simulink library "simplex_lib"  (R2020b)
settings: Solver=VariableStepAuto  StartTime=0.0  StopTime=10.0  RelTol=1e-3
values from neighbouring files (symbols this model uses):
  Ts = 1/Fs    [MainSimulink.m]
undefined symbols (not defined in the file or in its folder): ang_r, DiscIntNeverNeededParam, P_dc, Sbase, Tm_pu, Vbase, w0, Wbase, wbase
libraries: powerlib x62, $bdroot x14
settings Model: Creator=admin_user  LastModifiedBy=admin_user
settings DataIOCC: ReturnWorkspaceOutputs=off
settings DebuggingCC: ArithmeticOperatorsInVariantConditions=warning
settings SFSimCC: SimUseLocalCustomCode=off  CustomCodeUndefinedFunction=UseInterfaceOnly
settings RTWCC: RTWUseLocalCustomCode=off

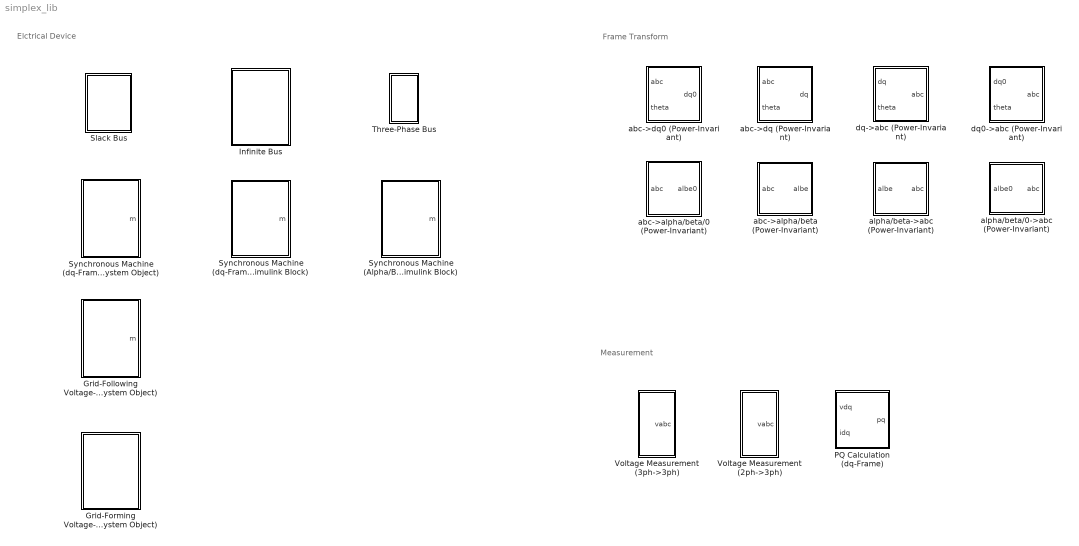
== system simplex_lib ==
  note: Elctrical Device
  note: Measurement
  note: Frame Transform
  Grid-Following Voltage-Source Inverter (dq-Frame System Object) : Subsystem  mask{Sbase=Sbase, Vbase=Vbase, Wbase=Wbase, Ts=Ts, DeviceType=10, DevicePara=[], PowerFlow=[], x0=[0; 0; 0; 0; 2.5*Vbase; 0; 0; Wbase; 0], OtherInputs=[ang_r; P_dc]}
      mask prompts: Ts "Ts (s)"
  Grid-Forming Voltage-Source Inverter (dq-Frame System Object) : Subsystem  mask{DeviceType=10, DevicePara=[], PowerFlow=[], theta0=0, ang_r=0, P_dc=0, Ts=Ts, x0=[0;0;0;0;1;0;0;0;0;0;w0;1]}
      mask prompts: Ts "Ts (s)"
  Infinite Bus : Subsystem  mask{Sbase=1, Vbase=1, Wbase=Wbase, Vdq0=[1,0,0], w=1, theta0=0}
      mask prompts: Sbase "Sbase (VA)"; Vbase "Vbase (V)"; Wbase "Wbase (rad/s)"; Vdq0 "Vdq0 (pu)"; w "w (pu)"; theta0 "theta0 (rad)"
  PQ Calculation (dq-Frame) : Subsystem  mask{wfil=wbase/10, Ts=Ts}
      mask prompts: wfil "Filter Bandwidth (rad/s)"; Ts "Sampling Time"
  Slack Bus : Subsystem  mask{vd=1, vq=0, v0=0, w=1, theta0=0, Vbase=Vbase, Wbase=Wbase}
      mask prompts: vd "vd (pu)"; vq "vq (pu)"; v0 "v0 (pu)"; w "w (pu)"; theta0 "theta0 (rad)"; Vbase "Vbase (V)"; Wbase "Wbase (rad/s)"
  Synchronous Machine (Alpha/Beta-Frame Simulink Block) : Subsystem  mask{Ts=Ts, Sbase=Sbase, Vbase=Vbase, Wbase=Wbase, R=0.01, L=0.3, J=2*3.5, D=10, psi_f=1.1229, Tm=-10.890, w0=1, theta0=0}
      mask prompts: Ts "Sampling Time, Ts (s)"; Sbase "Base Power, Sbase (VA)"; Vbase "Base Voltage, Vbase (V)"; Wbase "Base Angular Frequency, Wbase (rad/s)"; R "Stator Resistance, R (pu)"; L "Stator Inductance, L (pu)"; J "Rotor Inertia, J (pu)"; D "Damoing Torque Coefficient, D (pu)"; psi_f "Field Flux Linkage, psi_f (pu)"; Tm "Mechanical Torque, Tm (pu)"; w0 "Intial Value of Rotor Speed, w0 (pu)"; theta0 "Initial Value of Rotor Angle, theta0 (rad)"
  Synchronous Machine (dq-Frame Simulink Block) : Subsystem  mask{Ts=Ts, Sbase=Sbase, Vbase=Vbase, Wbase=Wbase, R=0.01, L=0.3, J=2*3.5, D=10, psi_f=1.1229, Tm=-10.890, w0=1, theta0=0}
      mask prompts: Ts "Sampling Time, Ts (s)"; Sbase "Base Power, Sbase (VA)"; Vbase "Base Voltage, Vbase (V)"; Wbase "Base Angular Frequency, Wbase (rad/s)"; R "Stator Resistance, R (pu)"; L "Stator Inductance, L (pu)"; J "Rotor Inertia, J (pu)"; D "Damping Torque Coefficient, D (pu)"; psi_f "Field Flux Linkage, psi_f"; Tm "Mechanical Torque, Tm (pu)"; w0 "Intial Rotor Speed, w0 (pu)"; theta0 "Initial Rotor Angle, theta0 (rad)"
  Synchronous Machine (dq-Frame System Object) : Subsystem  mask{Sbase=Sbase, Vbase=Vbase, Wbase=Wbase, Ts=Ts, DeviceType=0, DevicePara=[], PowerFlow=[], x0=[0;0;Wbase;0], OtherInputs=[Tm_pu/Wbase;0]}
      mask prompts: Sbase "Sbase (VA)"; Vbase "Vbase (V)"; Wbase "Wbase (rad/s)"; Ts "Ts (s)"
  Three-Phase Bus : Subsystem  mask{Vbase=1, Sbase=1}
  Voltage Measurement (2ph->3ph) : Subsystem
  Voltage Measurement (3ph->3ph) : Subsystem
  abc->alpha/beta (Power-Invariant) : Subsystem
  abc->alpha/beta/0 (Power-Invariant) : Subsystem
  abc->dq (Power-Invariant) : Subsystem
  abc->dq0 (Power-Invariant) : Subsystem
  alpha/beta->abc (Power-Invariant) : Subsystem
  alpha/beta/0->abc (Power-Invariant) : Subsystem
  dq->abc (Power-Invariant) : Subsystem
  dq0->abc (Power-Invariant) : Subsystem

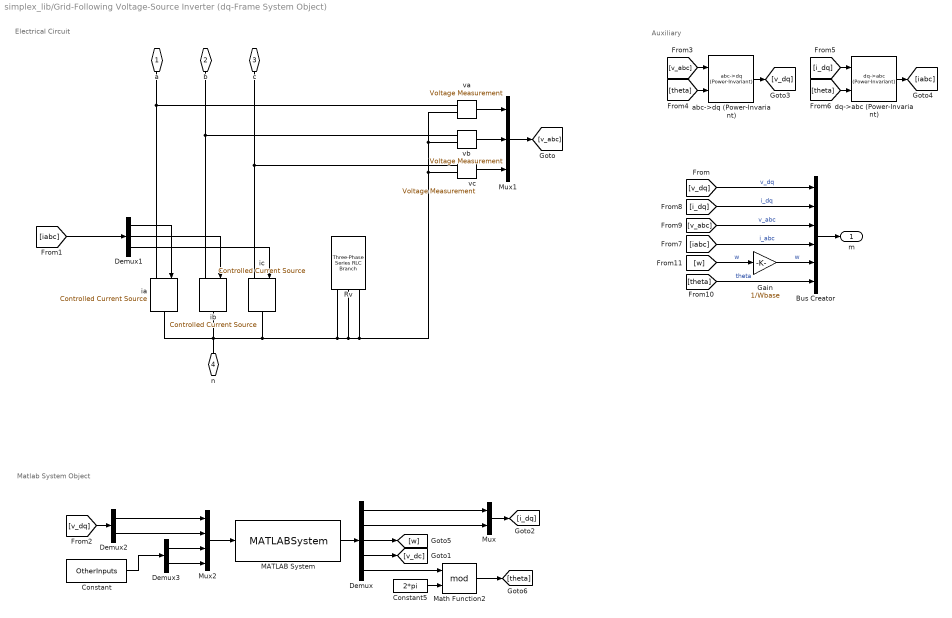
== system simplex_lib/Grid-Following Voltage-Source Inverter (dq-Frame System Object) ==
  note: Matlab System Object
  note: Auxiliary
  note: Electrical Circuit
  Bus Creator : BusCreator  Inputs=6
  Constant : Constant  Value=OtherInputs
  Constant5 : Constant  Value=2*pi
  Demux : Demux  Outputs=5
  Demux1 : Demux  Outputs=3
  Demux2 : Demux  Outputs=2
  Demux3 : Demux  Outputs=2
  Gain : Gain  Gain=1/Wbase
  MATLAB System : MATLABSystem  System=Class_GridFollowingVSI  DeviceType=DeviceType  Para=DevicePara  PowerFlow=PowerFlow  Ts=Ts  x0=x0  SimulateUsing=Code generation
      mask Type: Class_GridFollowingVSI
      mask Display:
      | disp('Class_GridFollowingVSI');
      | port_label('input',1,'u');
      | port_label('output',1,'y');
  Math Function2 : Math  Operator=mod  SignedPower=on  SaturateOnIntegerOverflow=on
  Mux : Mux  Inputs=2
  Mux1 : Mux  Inputs=3
  Mux2 : Mux
  Rv : powerlib/Elements/Three-Phase Series RLC Branch  LConnTagsString=A|B|C  RConnTagsString=A|B|C  BranchType=R  Resistance=2*DevicePara(3)/Ts  Inductance=1e-3  Capacitance=1e-6  Measurements=None
  abc->dq (Power-Invariant) : $bdroot/abc->dq (Power-Invariant)  SystemSampleTime=-1  VariantActivationTime=update diagram  Latency=0  AutoFrameSizeCalculation=off
  dq->abc (Power-Invariant) : $bdroot/dq->abc (Power-Invariant)  SystemSampleTime=-1  VariantActivationTime=update diagram  Latency=0  AutoFrameSizeCalculation=off
  ia : powerlib/Electrical Sources/Controlled Current Source  Initialize=on  Source_Type=AC  Amplitude=0  Phase=0  Frequency=0  Measurements=None
  ib : powerlib/Electrical Sources/Controlled Current Source  Initialize=on  Source_Type=AC  Amplitude=0  Phase=0  Frequency=0  Measurements=None
  ic : powerlib/Electrical Sources/Controlled Current Source  Initialize=on  Source_Type=AC  Amplitude=0  Phase=0  Frequency=0  Measurements=None
  va : powerlib/Measurements/Voltage Measurement  PhasorSimulation=off  OutputType=Complex  PSBequivalent=0
  vb : powerlib/Measurements/Voltage Measurement  PhasorSimulation=off  OutputType=Complex  PSBequivalent=0
  vc : powerlib/Measurements/Voltage Measurement  PhasorSimulation=off  OutputType=Complex  PSBequivalent=0
  a : PMIOPort  Side=Left
  b : PMIOPort  Port=2  Side=Left
  c : PMIOPort  Port=3  Side=Left
  n : PMIOPort  Port=4  Side=Left
  m : Outport
  wires:
  Demux/2 -> Mux/2
  Demux/1 -> Mux/1
  Mux/1 -> [i_dq]
  Demux/3 -> [w]
  Demux1/1 -> ia/1
  Demux1/2 -> ib/1
  va/1 -> Mux1/1
  vb/1 -> Mux1/2
  Mux1/1 -> [v_abc]
  [v_dq] -> Demux2/1
  Demux2/1 -> Mux2/1
  Demux2/2 -> Mux2/2
  [v_dq] -> Bus Creator/1  "v_dq"
  [i_dq] -> Bus Creator/2  "i_dq"
  [v_abc] -> Bus Creator/3  "v_abc"
  [iabc] -> Bus Creator/4  "i_abc"
  [theta] -> Bus Creator/6  "theta"
  [v_abc] -> abc->dq (Power-Invariant)/1
  [theta] -> abc->dq (Power-Invariant)/2
  abc->dq (Power-Invariant)/1 -> [v_dq]
  [i_dq] -> dq->abc (Power-Invariant)/1
  [theta] -> dq->abc (Power-Invariant)/2
  dq->abc (Power-Invariant)/1 -> [iabc]
  Mux2/1 -> MATLAB System/1
  MATLAB System/1 -> Demux/1
  vc/1 -> Mux1/3
  Demux1/3 -> ic/1
  Demux/5 -> Math Function2/1
  Constant5/1 -> Math Function2/2
  Math Function2/1 -> [theta]
  Demux/4 -> [v_dc]
  Bus Creator/1 -> m/1
  Demux3/1 -> Mux2/3
  Demux3/2 -> Mux2/4
  Constant/1 -> Demux3/1
  [w] -> Gain/1  "w"
  Gain/1 -> Bus Creator/5  "w"
  [iabc] -> Demux1/1
  connections:
  vb/LConn2 -- va/LConn2 -- vc/LConn2 -- Rv/RConn3 -- Rv/RConn2 -- Rv/RConn1 -- ic/RConn1 -- ia/RConn1 -- ib/RConn1 -- n/RConn1
  a/RConn1 -- ia/LConn1 -- va/LConn1
  b/RConn1 -- vb/LConn1 -- ib/LConn1
  vc/LConn1 -- ic/LConn1 -- c/RConn1

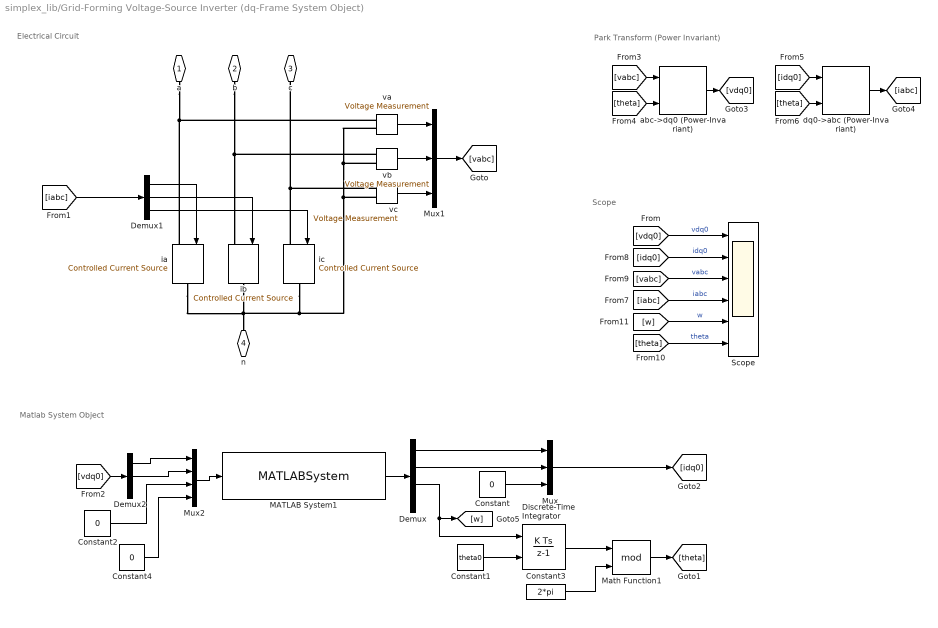
== system simplex_lib/Grid-Forming Voltage-Source Inverter (dq-Frame System Object) ==
  note: Scope
  note: Matlab System Object
  note: Park Transform (Power Invariant)
  note: Electrical Circuit
  Constant : Constant  Value=0
  Constant1 : Constant  Value=theta0
  Constant2 : Constant  Value=0
  Constant3 : Constant  Value=2*pi
  Constant4 : Constant  Value=0
  Demux : Demux
  Demux1 : Demux  Outputs=3
  Demux2 : Demux  Outputs=3
  Discrete-Time Integrator : DiscreteIntegrator  InitialConditionSource=external  SampleTime=Ts  ICPrevOutput=DiscIntNeverNeededParam  ICPrevScaledInput=DiscIntNeverNeededParam
  MATLAB System1 : MATLABSystem  System=Class_GridFormingVSI  DeviceType=DeviceType  Para=DevicePara  PowerFlow=PowerFlow  Ts=Ts  x0=x0  SimulateUsing=Code generation
      mask Type: Class_GridFormingVSI
      mask Display:
      | disp('Class_GridFormingVSI');
      | port_label('input',1,'u');
      | port_label('output',1,'y');
  Math Function1 : Math  Operator=mod  SignedPower=on  SaturateOnIntegerOverflow=on
  Mux : Mux  Inputs=3
  Mux1 : Mux  Inputs=3
  Mux2 : Mux
  Scope : Scope  NumInputPorts=6
  abc->dq0 (Power-Invariant) : $bdroot/abc->dq0 (Power-Invariant)  SystemSampleTime=-1  VariantActivationTime=update diagram  Latency=0  AutoFrameSizeCalculation=off
  dq0->abc (Power-Invariant) : $bdroot/dq0->abc (Power-Invariant)  SystemSampleTime=-1  VariantActivationTime=update diagram  Latency=0  AutoFrameSizeCalculation=off
  ia : powerlib/Electrical Sources/Controlled Current Source  Initialize=on  Source_Type=AC  Amplitude=0  Phase=0  Frequency=0  Measurements=None
  ib : powerlib/Electrical Sources/Controlled Current Source  Initialize=on  Source_Type=AC  Amplitude=0  Phase=0  Frequency=0  Measurements=None
  ic : powerlib/Electrical Sources/Controlled Current Source  Initialize=on  Source_Type=AC  Amplitude=0  Phase=0  Frequency=0  Measurements=None
  va : powerlib/Measurements/Voltage Measurement  PhasorSimulation=off  OutputType=Complex  PSBequivalent=0
  vb : powerlib/Measurements/Voltage Measurement  PhasorSimulation=off  OutputType=Complex  PSBequivalent=0
  vc : powerlib/Measurements/Voltage Measurement  PhasorSimulation=off  OutputType=Complex  PSBequivalent=0
  a : PMIOPort  Side=Left
  b : PMIOPort  Port=2  Side=Left
  c : PMIOPort  Port=3  Side=Left
  n : PMIOPort  Port=4  Side=Left
  wires:
  Constant/1 -> Mux/3
  Demux/2 -> Mux/2
  Demux/1 -> Mux/1
  Mux/1 -> [idq0]
  Demux/3 -> Discrete-Time Integrator/1, [w]
  Constant1/1 -> Discrete-Time Integrator/2
  Demux1/1 -> ia/1
  Demux1/2 -> ib/1
  va/1 -> Mux1/1
  vb/1 -> Mux1/2
  Mux1/1 -> [vabc]
  [vdq0] -> Demux2/1
  Demux2/1 -> Mux2/1
  Demux2/2 -> Mux2/2
  Constant3/1 -> Math Function1/2
  Discrete-Time Integrator/1 -> Math Function1/1
  Math Function1/1 -> [theta]
  [vdq0] -> Scope/1  "vdq0"
  [idq0] -> Scope/2  "idq0"
  [vabc] -> Scope/3  "vabc"
  [iabc] -> Scope/4  "iabc"
  [w] -> Scope/5  "w"
  [theta] -> Scope/6  "theta"
  [vabc] -> abc->dq0 (Power-Invariant)/1
  [theta] -> abc->dq0 (Power-Invariant)/2
  abc->dq0 (Power-Invariant)/1 -> [vdq0]
  [idq0] -> dq0->abc (Power-Invariant)/1
  [theta] -> dq0->abc (Power-Invariant)/2
  dq0->abc (Power-Invariant)/1 -> [iabc]
  Mux2/1 -> MATLAB System1/1
  MATLAB System1/1 -> Demux/1
  vc/1 -> Mux1/3
  Demux1/3 -> ic/1
  [iabc] -> Demux1/1
  Constant2/1 -> Mux2/3
  Constant4/1 -> Mux2/4
  connections:
  vb/LConn2 -- va/LConn2 -- vc/LConn2 -- ic/RConn1 -- ia/RConn1 -- ib/RConn1 -- n/RConn1
  a/RConn1 -- ia/LConn1 -- va/LConn1
  b/RConn1 -- vb/LConn1 -- ib/LConn1
  vc/LConn1 -- ic/LConn1 -- c/RConn1

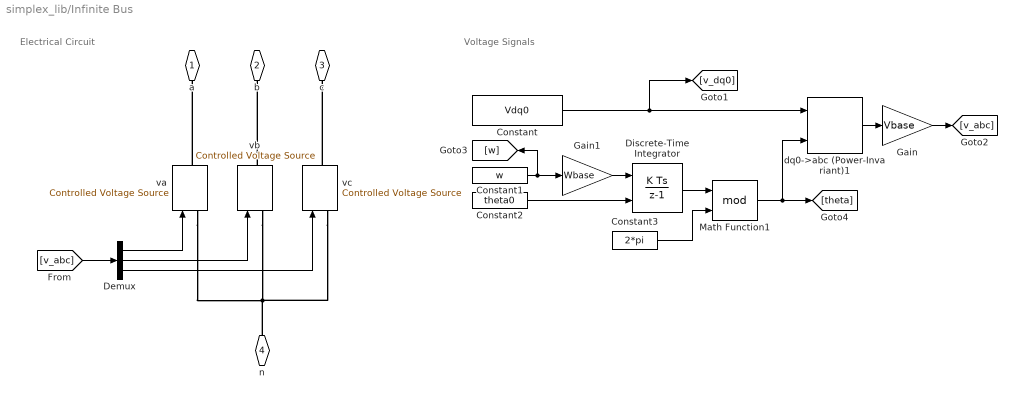
== system simplex_lib/Infinite Bus ==
  note: Voltage Signals
  note: Electrical Circuit
  Constant : Constant  Value=Vdq0
  Constant1 : Constant  Value=w
  Constant2 : Constant  Value=theta0
  Constant3 : Constant  Value=2*pi
  Demux : Demux  Outputs=3
  Discrete-Time Integrator : DiscreteIntegrator  InitialConditionSource=external  SampleTime=Ts  ICPrevOutput=DiscIntNeverNeededParam  ICPrevScaledInput=DiscIntNeverNeededParam
  Gain : Gain  Gain=Vbase
  Gain1 : Gain  Gain=Wbase
  Math Function1 : Math  Operator=mod  SignedPower=on  SaturateOnIntegerOverflow=on
  dq0->abc (Power-Invariant)1 : $bdroot/dq0->abc (Power-Invariant)  SystemSampleTime=-1  VariantActivationTime=update diagram  Latency=0  AutoFrameSizeCalculation=off
  va : powerlib/Electrical Sources/Controlled Voltage Source  Initialize=on  Source_Type=AC  Amplitude=0  Phase=0  Frequency=0  Measurements=None
  vb : powerlib/Electrical Sources/Controlled Voltage Source  Initialize=on  Source_Type=AC  Amplitude=0  Phase=0  Frequency=0  Measurements=None
  vc : powerlib/Electrical Sources/Controlled Voltage Source  Initialize=on  Source_Type=AC  Amplitude=0  Phase=0  Frequency=0  Measurements=None
  a : PMIOPort  Side=Right
  b : PMIOPort  Port=2  Side=Right
  c : PMIOPort  Port=3  Side=Right
  n : PMIOPort  Port=4  Side=Right
  wires:
  Constant1/1 -> [w], Gain1/1
  Constant/1 -> dq0->abc (Power-Invariant)1/1, [v_dq0]
  Constant2/1 -> Discrete-Time Integrator/2
  Constant3/1 -> Math Function1/2
  Math Function1/1 -> dq0->abc (Power-Invariant)1/2, [theta]
  Demux/1 -> va/1
  [v_abc] -> Demux/1
  Demux/2 -> vb/1
  Gain/1 -> [v_abc]
  Gain1/1 -> Discrete-Time Integrator/1
  Discrete-Time Integrator/1 -> Math Function1/1
  Demux/3 -> vc/1
  dq0->abc (Power-Invariant)1/1 -> Gain/1
  connections:
  vb/RConn1 -- b/RConn1
  va/RConn1 -- a/RConn1
  vc/LConn1 -- n/RConn1 -- va/LConn1 -- vb/LConn1
  vc/RConn1 -- c/RConn1

== system simplex_lib/PQ Calculation (dq-Frame) ==
  vdq : Inport
  idq : Inport  Port=2
  Mux : Mux  Inputs=2
  Mux1 : Mux  Inputs=2
  P = vd*id+vq*iq : Fcn  Expr=u[1]*u[3]+u[2]*u[4]
  Q = -vd*iq+vq*id : Fcn  Expr=-u[1]*u[4]+u[2]*u[3]
  pq : Outport  VectorParamsAs1DForOutWhenUnconnected=off
  wires:
  Q = -vd*iq+vq*id/1 -> Mux/2
  Mux1/1 -> Q = -vd*iq+vq*id/1, P = vd*id+vq*iq/1
  idq/1 -> Mux1/2
  vdq/1 -> Mux1/1
  P = vd*id+vq*iq/1 -> Mux/1
  Mux/1 -> pq/1

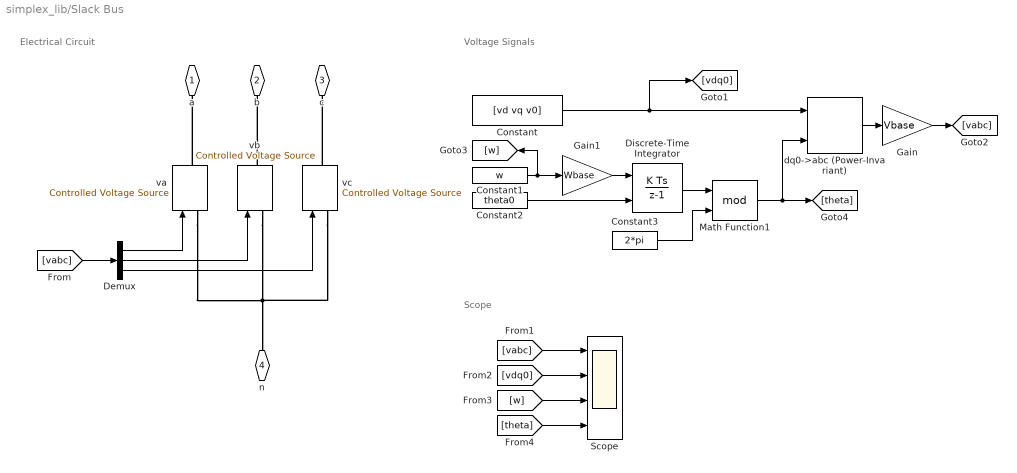
== system simplex_lib/Slack Bus ==
  note: Scope
  note: Voltage Signals
  note: Electrical Circuit
  Constant : Constant  Value=[vd vq v0]
  Constant1 : Constant  Value=w
  Constant2 : Constant  Value=theta0
  Constant3 : Constant  Value=2*pi
  Demux : Demux  Outputs=3
  Discrete-Time Integrator : DiscreteIntegrator  InitialConditionSource=external  SampleTime=Ts  ICPrevOutput=DiscIntNeverNeededParam  ICPrevScaledInput=DiscIntNeverNeededParam
  Gain : Gain  Gain=Vbase
  Gain1 : Gain  Gain=Wbase
  Math Function1 : Math  Operator=mod  SignedPower=on  SaturateOnIntegerOverflow=on
  Scope : Scope  NumInputPorts=4
  dq0->abc (Power-Invariant) : $bdroot/dq0->abc (Power-Invariant)  SystemSampleTime=-1  VariantActivationTime=update diagram  Latency=0  AutoFrameSizeCalculation=off
  va : powerlib/Electrical Sources/Controlled Voltage Source  Initialize=on  Source_Type=AC  Amplitude=0  Phase=0  Frequency=0  Measurements=None
  vb : powerlib/Electrical Sources/Controlled Voltage Source  Initialize=on  Source_Type=AC  Amplitude=0  Phase=0  Frequency=0  Measurements=None
  vc : powerlib/Electrical Sources/Controlled Voltage Source  Initialize=on  Source_Type=AC  Amplitude=0  Phase=0  Frequency=0  Measurements=None
  a : PMIOPort  Side=Right
  b : PMIOPort  Port=2  Side=Right
  c : PMIOPort  Port=3  Side=Right
  n : PMIOPort  Port=4  Side=Left
  wires:
  Constant/1 -> dq0->abc (Power-Invariant)/1, [vdq0]
  Constant2/1 -> Discrete-Time Integrator/2
  Constant1/1 -> [w], Gain1/1
  dq0->abc (Power-Invariant)/1 -> Gain/1
  Gain/1 -> [vabc]
  [vabc] -> Demux/1
  Demux/1 -> va/1
  Demux/2 -> vb/1
  Demux/3 -> vc/1
  Gain1/1 -> Discrete-Time Integrator/1
  [vabc] -> Scope/1
  [vdq0] -> Scope/2
  [w] -> Scope/3
  Constant3/1 -> Math Function1/2
  Discrete-Time Integrator/1 -> Math Function1/1
  Math Function1/1 -> dq0->abc (Power-Invariant)/2, [theta]
  [theta] -> Scope/4
  connections:
  vc/RConn1 -- c/RConn1
  va/RConn1 -- a/RConn1
  vb/RConn1 -- b/RConn1
  va/LConn1 -- vb/LConn1 -- vc/LConn1 -- n/RConn1

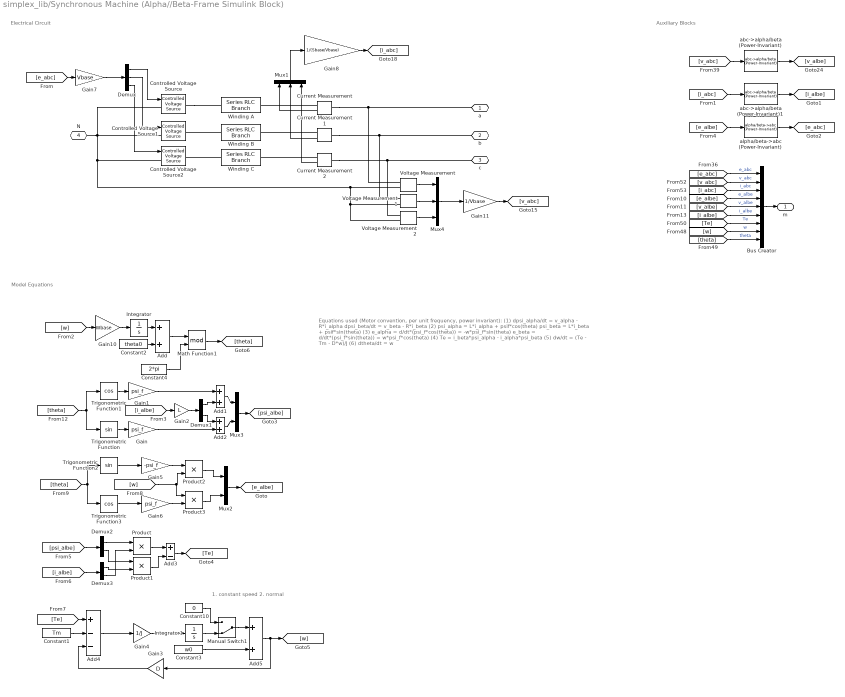
== system simplex_lib/Synchronous Machine (Alpha//Beta-Frame Simulink Block) ==
  note: 1. constant speed
      | 2. normal
  note: Auxiliary Blocks
  note: Model Equations
  note: Electrical Circuit
  note: Equations used
      | (Motor convention, per unit frequency, power invariant):
      |
      | (1) dpsi_alpha/dt = v_alpha - R*i_alpha
      | dpsi_beta/dt = v_beta - R*i_beta
      |
      | (2) psi_alpha = L*i_alpha + psif*cos(theta)
      | psi_beta = L*i_beta + psif*sin(theta)
      |
      | (3) e_alpha = d/dt*(psi_f*cos(theta)) = -w*psi_f*sin(theta)
      | e_beta = d/dt*(psi_f*sin(theta)) = w*psi_f*cos(theta)
      |
      | (4) Te = i_beta*psi_alpha - i_alpha*psi_beta
      | (5) dw/dt = (Te - Tm - D*w)/J
      | (6) dtheta/dt = w
  Add{,1..2,5} (4 alike) : Sum
  Add3 : Sum  Inputs=+-
  Add4 : Sum  Inputs=+--
  Bus Creator : BusCreator  Inputs=9
  Constant1 : Constant  Value=Tm
  Constant10 : Constant  Value=0
  Constant2 : Constant  Value=theta0
  Constant3 : Constant  Value=w0
  Constant4 : Constant  Value=2*pi
  Controlled Voltage Source : powerlib/Electrical Sources/Controlled Voltage Source  Initialize=on  Source_Type=AC  Amplitude=0  Phase=0  Frequency=0  Measurements=None
  Controlled Voltage Source1 : powerlib/Electrical Sources/Controlled Voltage Source  Initialize=on  Source_Type=AC  Amplitude=0  Phase=0  Frequency=0  Measurements=None
  Controlled Voltage Source2 : powerlib/Electrical Sources/Controlled Voltage Source  Initialize=on  Source_Type=AC  Amplitude=0  Phase=0  Frequency=0  Measurements=None
  Current Measurement : powerlib/Measurements/Current Measurement  PhasorSimulation=off  OutputType=Complex  PSBequivalent=0
  Current Measurement1 : powerlib/Measurements/Current Measurement  PhasorSimulation=off  OutputType=Complex  PSBequivalent=0
  Current Measurement2 : powerlib/Measurements/Current Measurement  PhasorSimulation=off  OutputType=Complex  PSBequivalent=0
  Demux : Demux  Outputs=3
  Demux1 : Demux  Outputs=2
  Demux2 : Demux  Outputs=2
  Demux3 : Demux  Outputs=2
  Gain : Gain  Gain=psi_f
  Gain1 : Gain  Gain=psi_f
  Gain10 : Gain  Gain=Wbase
  Gain11 : Gain  Gain=1/Vbase
  Gain2 : Gain  Gain=L
  Gain3 : Gain  Gain=D
  Gain4 : Gain  Gain=1/J
  Gain5 : Gain  Gain=-psi_f
  Gain6 : Gain  Gain=psi_f
  Gain7 : Gain  Gain=Vbase
  Gain8 : Gain  Gain=1/(Sbase/Vbase)
  Integrator : Integrator
  Integrator1 : Integrator
  Manual Switch1 : ManualSwitch  CurrentSetting=0
  Math Function1 : Math  Operator=mod  SignedPower=on  SaturateOnIntegerOverflow=on
  Mux1 : Mux  Inputs=3
  Mux2 : Mux  Inputs=2
  Mux3 : Mux  Inputs=2
  Mux4 : Mux  Inputs=3
  Product{,1..3} (4 alike) : Product
  Trigonometric Function : Trigonometry
  Trigonometric Function1 : Trigonometry  Operator=cos
  Trigonometric Function2 : Trigonometry
  Trigonometric Function3 : Trigonometry  Operator=cos
  Voltage Measurement : powerlib/Measurements/Voltage Measurement  PhasorSimulation=off  OutputType=Complex  PSBequivalent=0
  Voltage Measurement1 : powerlib/Measurements/Voltage Measurement  PhasorSimulation=off  OutputType=Complex  PSBequivalent=0
  Voltage Measurement2 : powerlib/Measurements/Voltage Measurement  PhasorSimulation=off  OutputType=Complex  PSBequivalent=0
  Winding A : powerlib/Elements/Series RLC Branch  LConnTagsString=__new0  RConnTagsString=__new0  BranchType=RL  Resistance=R*(Vbase^2)/Sbase  Inductance=L*(Vbase^2)/Sbase/Wbase  SetiL0=off  InitialCurrent=ia0  Capacitance=1e-6  Setx0=off  InitialVoltage=0  Measurements=None
  Winding B : powerlib/Elements/Series RLC Branch  LConnTagsString=__new0  RConnTagsString=__new0  BranchType=RL  Resistance=R*(Vbase^2)/Sbase  Inductance=L*(Vbase^2)/Sbase/Wbase  SetiL0=off  InitialCurrent=ia0  Capacitance=1e-6  Setx0=off  InitialVoltage=0  Measurements=None
  Winding C : powerlib/Elements/Series RLC Branch  LConnTagsString=__new0  RConnTagsString=__new0  BranchType=RL  Resistance=R*(Vbase^2)/Sbase  Inductance=L*(Vbase^2)/Sbase/Wbase  SetiL0=off  InitialCurrent=ia0  Capacitance=1e-6  Setx0=off  InitialVoltage=0  Measurements=None
  abc->alpha/beta (Power-Invariant) : $bdroot/abc->alpha//beta (Power-Invariant)  SystemSampleTime=-1  VariantActivationTime=update diagram  Latency=0  AutoFrameSizeCalculation=off
  abc->alpha/beta (Power-Invariant)1 : $bdroot/abc->alpha//beta (Power-Invariant)  SystemSampleTime=-1  VariantActivationTime=update diagram  Latency=0  AutoFrameSizeCalculation=off
  alpha/beta->abc (Power-Invariant) : $bdroot/alpha//beta->abc (Power-Invariant)  SystemSampleTime=-1  VariantActivationTime=update diagram  Latency=0  AutoFrameSizeCalculation=off
  a : PMIOPort  Side=Left
  b : PMIOPort  Port=2  Side=Left
  c : PMIOPort  Port=3  Side=Left
  N : PMIOPort  Port=4  Side=Left
  m : Outport
  wires:
  Current Measurement/1 -> Mux1/1
  Current Measurement1/1 -> Mux1/2
  Current Measurement2/1 -> Mux1/3
  Mux1/1 -> Gain8/1
  [e_abc] -> Gain7/1
  Demux/1 -> Controlled Voltage Source/1
  Demux/2 -> Controlled Voltage Source1/1
  Demux/3 -> Controlled Voltage Source2/1
  [i_abc] -> abc->alpha/beta (Power-Invariant)1/1
  abc->alpha/beta (Power-Invariant)1/1 -> [i_albe]
  [w] -> Gain10/1
  Integrator/1 -> Add/1
  Constant2/1 -> Add/2
  Trigonometric Function1/1 -> Gain1/1
  Trigonometric Function/1 -> Gain/1
  [i_albe] -> Gain2/1
  Demux1/1 -> Add1/2
  Demux1/2 -> Add2/1
  Gain2/1 -> Demux1/1
  Gain1/1 -> Add1/1
  Gain/1 -> Add2/2
  Product2/1 -> Mux2/1
  Product3/1 -> Mux2/2
  Mux2/1 -> [e_albe]
  [e_albe] -> alpha/beta->abc (Power-Invariant)/1
  alpha/beta->abc (Power-Invariant)/1 -> [e_abc]
  Add1/1 -> Mux3/1
  Add2/1 -> Mux3/2
  Mux3/1 -> [psi_albe]
  [psi_albe] -> Demux2/1
  [i_albe] -> Demux3/1
  Demux2/1 -> Product/1
  Demux3/2 -> Product/2
  Demux3/1 -> Product1/2
  Demux2/2 -> Product1/1
  Product/1 -> Add3/1
  Product1/1 -> Add3/2
  Add3/1 -> [Te]
  [Te] -> Add4/1
  Constant1/1 -> Add4/2
  Add4/1 -> Gain4/1
  Gain3/1 -> Add4/3
  Constant3/1 -> Add5/2
  Add5/1 -> Gain3/1, [w]
  [theta] -> Trigonometric Function3/1, Trigonometric Function2/1
  Trigonometric Function2/1 -> Gain5/1
  Trigonometric Function3/1 -> Gain6/1
  Gain5/1 -> Product2/1
  Gain6/1 -> Product3/2
  Gain8/1 -> [i_abc]
  Gain4/1 -> Integrator1/1
  Gain10/1 -> Integrator/1
  Voltage Measurement/1 -> Mux4/1
  Voltage Measurement1/1 -> Mux4/2
  Voltage Measurement2/1 -> Mux4/3
  Mux4/1 -> Gain11/1
  Gain11/1 -> [v_abc]
  Gain7/1 -> Demux/1
  Add/1 -> Math Function1/1
  Constant4/1 -> Math Function1/2
  Math Function1/1 -> [theta]
  [v_abc] -> abc->alpha/beta (Power-Invariant)/1
  abc->alpha/beta (Power-Invariant)/1 -> [v_albe]
  [w] -> Product3/1, Product2/2
  [theta] -> Trigonometric Function/1, Trigonometric Function1/1
  Integrator1/1 -> Manual Switch1/2
  Manual Switch1/1 -> Add5/1
  Constant10/1 -> Manual Switch1/1
  [e_abc] -> Bus Creator/1  "e_abc"
  [v_abc] -> Bus Creator/2  "v_abc"
  [i_abc] -> Bus Creator/3  "i_abc"
  [e_albe] -> Bus Creator/4  "e_albe"
  [v_albe] -> Bus Creator/5  "v_albe"
  [i_albe] -> Bus Creator/6  "i_albe"
  [Te] -> Bus Creator/7  "Te"
  [w] -> Bus Creator/8  "w"
  [theta] -> Bus Creator/9  "theta"
  Bus Creator/1 -> m/1
  connections:
  Current Measurement/RConn1 -- Winding A/RConn1
  Controlled Voltage Source/RConn1 -- Winding A/LConn1
  Current Measurement2/RConn1 -- Winding C/RConn1
  Current Measurement/LConn1 -- Voltage Measurement/LConn1 -- a/RConn1
  Current Measurement1/LConn1 -- Voltage Measurement1/LConn1 -- b/RConn1
  Current Measurement1/RConn1 -- Winding B/RConn1
  Winding B/LConn1 -- Controlled Voltage Source1/RConn1
  Controlled Voltage Source/LConn1 -- Voltage Measurement2/LConn2 -- Voltage Measurement1/LConn2 -- Voltage Measurement/LConn2 -- Controlled Voltage Source2/LConn1 -- N/RConn1 -- Controlled Voltage Source1/LConn1
  Winding C/LConn1 -- Controlled Voltage Source2/RConn1
  Current Measurement2/LConn1 -- Voltage Measurement2/LConn1 -- c/RConn1

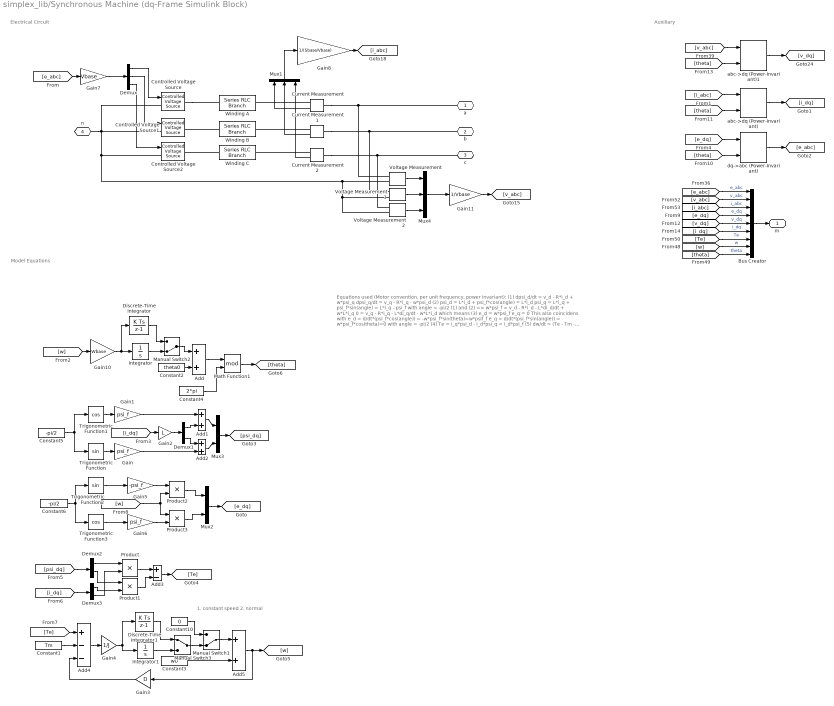
== system simplex_lib/Synchronous Machine (dq-Frame Simulink Block) ==
  note: 1. constant speed
      | 2. normal
  note: Auxiliary
  note: Model Equations
  note: Electrical Circuit
  note: Equations used
      | (Motor convention, per unit frequency, power invariant):
      |
      | (1) dpsi_d/dt = v_d - R*i_d + w*psi_q
      | dpsi_q/dt = v_q - R*i_q - w*psi_d
      |
      | (2) psi_d = L*i_d + psi_f*cos(angle) = L*i_d
      | psi_q = L*i_q + psi_f*sin(angle) = L*i_q - psi_f
      | with angle = -pi/2
      |
      | (1) and (2) =>
      |
      | w*psi_f = v_d - R*i_d - L*di_d/dt + w*L*i_q
      | 0 = v_q - R*i_q - L*di_q/dt - w*L*i_d
      |
      | which means
      |
      | (3) e_d = w*psi_f
      | e_q = 0
      |
      | This also coincidens with
      |
      | e_d = d/dt*(psi_f*cos(angle)) = -w*psi_f*sin(theta)=w*psif_f
      | e_q = d/dt*(psi_f*sin(angle)) = w*psi_f*cos(theta)=0
      | with angle = -pi/2
      |
      | (4) Te = i_q*psi_d - i_d*psi_q = i_d*psi_f
      | (5) dw/dt = (Te - Tm - D*w)/J
      | (6) dtheta/dt = w
  Add{,1..2,5} (4 alike) : Sum
  Add3 : Sum  Inputs=+-
  Add4 : Sum  Inputs=+--
  Bus Creator : BusCreator  Inputs=9
  Constant1 : Constant  Value=Tm
  Constant10 : Constant  Value=0
  Constant2 : Constant  Value=theta0
  Constant3 : Constant  Value=w0
  Constant4 : Constant  Value=2*pi
  Constant5 : Constant  Value=-pi/2
  Constant6 : Constant  Value=-pi/2
  Controlled Voltage Source : powerlib/Electrical Sources/Controlled Voltage Source  Initialize=on  Source_Type=AC  Amplitude=0  Phase=0  Frequency=0  Measurements=None
  Controlled Voltage Source1 : powerlib/Electrical Sources/Controlled Voltage Source  Initialize=on  Source_Type=AC  Amplitude=0  Phase=0  Frequency=0  Measurements=None
  Controlled Voltage Source2 : powerlib/Electrical Sources/Controlled Voltage Source  Initialize=on  Source_Type=AC  Amplitude=0  Phase=0  Frequency=0  Measurements=None
  Current Measurement : powerlib/Measurements/Current Measurement  PhasorSimulation=off  OutputType=Complex  PSBequivalent=0
  Current Measurement1 : powerlib/Measurements/Current Measurement  PhasorSimulation=off  OutputType=Complex  PSBequivalent=0
  Current Measurement2 : powerlib/Measurements/Current Measurement  PhasorSimulation=off  OutputType=Complex  PSBequivalent=0
  Demux : Demux  Outputs=3
  Demux1 : Demux  Outputs=2
  Demux2 : Demux  Outputs=2
  Demux3 : Demux  Outputs=2
  Discrete-Time Integrator : DiscreteIntegrator  SampleTime=-1  ICPrevOutput=DiscIntNeverNeededParam  ICPrevScaledInput=DiscIntNeverNeededParam
  Discrete-Time Integrator1 : DiscreteIntegrator  SampleTime=-1  ICPrevOutput=DiscIntNeverNeededParam  ICPrevScaledInput=DiscIntNeverNeededParam
  Gain : Gain  Gain=psi_f
  Gain1 : Gain  Gain=psi_f
  Gain10 : Gain  Gain=Wbase
  Gain11 : Gain  Gain=1/Vbase
  Gain2 : Gain  Gain=L
  Gain3 : Gain  Gain=D
  Gain4 : Gain  Gain=1/J
  Gain5 : Gain  Gain=-psi_f
  Gain6 : Gain  Gain=psi_f
  Gain7 : Gain  Gain=Vbase
  Gain8 : Gain  Gain=1/(Sbase/Vbase)
  Integrator : Integrator
  Integrator1 : Integrator
  Manual Switch1 : ManualSwitch  CurrentSetting=0
  Manual Switch2 : ManualSwitch  CurrentSetting=0
  Manual Switch3 : ManualSwitch
  Math Function1 : Math  Operator=mod  SignedPower=on  SaturateOnIntegerOverflow=on
  Mux1 : Mux  Inputs=3
  Mux2 : Mux  Inputs=2
  Mux3 : Mux  Inputs=2
  Mux4 : Mux  Inputs=3
  Product{,1..3} (4 alike) : Product
  Trigonometric Function : Trigonometry
  Trigonometric Function1 : Trigonometry  Operator=cos
  Trigonometric Function2 : Trigonometry
  Trigonometric Function3 : Trigonometry  Operator=cos
  Voltage Measurement : powerlib/Measurements/Voltage Measurement  PhasorSimulation=off  OutputType=Complex  PSBequivalent=0
  Voltage Measurement1 : powerlib/Measurements/Voltage Measurement  PhasorSimulation=off  OutputType=Complex  PSBequivalent=0
  Voltage Measurement2 : powerlib/Measurements/Voltage Measurement  PhasorSimulation=off  OutputType=Complex  PSBequivalent=0
  Winding A : powerlib/Elements/Series RLC Branch  LConnTagsString=__new0  RConnTagsString=__new0  BranchType=RL  Resistance=R*(Vbase^2)/Sbase  Inductance=L*(Vbase^2)/Sbase/Wbase  SetiL0=off  InitialCurrent=ia0  Capacitance=1e-6  Setx0=off  InitialVoltage=0  Measurements=None
  Winding B : powerlib/Elements/Series RLC Branch  LConnTagsString=__new0  RConnTagsString=__new0  BranchType=RL  Resistance=R*(Vbase^2)/Sbase  Inductance=L*(Vbase^2)/Sbase/Wbase  SetiL0=off  InitialCurrent=ia0  Capacitance=1e-6  Setx0=off  InitialVoltage=0  Measurements=None
  Winding C : powerlib/Elements/Series RLC Branch  LConnTagsString=__new0  RConnTagsString=__new0  BranchType=RL  Resistance=R*(Vbase^2)/Sbase  Inductance=L*(Vbase^2)/Sbase/Wbase  SetiL0=off  InitialCurrent=ia0  Capacitance=1e-6  Setx0=off  InitialVoltage=0  Measurements=None
  abc->dq (Power-Invariant) : $bdroot/abc->dq (Power-Invariant)  SystemSampleTime=-1  VariantActivationTime=update diagram  Latency=0  AutoFrameSizeCalculation=off
  abc->dq (Power-Invariant)1 : $bdroot/abc->dq (Power-Invariant)  SystemSampleTime=-1  VariantActivationTime=update diagram  Latency=0  AutoFrameSizeCalculation=off
  dq->abc (Power-Invariant) : $bdroot/dq->abc (Power-Invariant)  SystemSampleTime=-1  VariantActivationTime=update diagram  Latency=0  AutoFrameSizeCalculation=off
  a : PMIOPort  Side=Left
  b : PMIOPort  Port=2  Side=Left
  c : PMIOPort  Port=3  Side=Left
  n : PMIOPort  Port=4  Side=Left
  m : Outport
  wires:
  Current Measurement/1 -> Mux1/1
  Current Measurement1/1 -> Mux1/2
  Current Measurement2/1 -> Mux1/3
  Mux1/1 -> Gain8/1
  [e_abc] -> Gain7/1
  Demux/1 -> Controlled Voltage Source/1
  Demux/2 -> Controlled Voltage Source1/1
  Demux/3 -> Controlled Voltage Source2/1
  [i_abc] -> abc->dq (Power-Invariant)/1
  abc->dq (Power-Invariant)/1 -> [i_dq]
  [w] -> Gain10/1
  Constant2/1 -> Add/2
  Trigonometric Function1/1 -> Gain1/1
  Trigonometric Function/1 -> Gain/1
  [i_dq] -> Gain2/1
  Demux1/1 -> Add1/2
  Demux1/2 -> Add2/1
  Gain2/1 -> Demux1/1
  Gain1/1 -> Add1/1
  Gain/1 -> Add2/2
  Product2/1 -> Mux2/1
  Product3/1 -> Mux2/2
  Mux2/1 -> [e_dq]
  [e_dq] -> dq->abc (Power-Invariant)/1
  Add1/1 -> Mux3/1
  Add2/1 -> Mux3/2
  Mux3/1 -> [psi_dq]
  [psi_dq] -> Demux2/1
  [i_dq] -> Demux3/1
  Demux2/1 -> Product/1
  Demux3/2 -> Product/2
  Demux3/1 -> Product1/2
  Demux2/2 -> Product1/1
  Product/1 -> Add3/1
  Product1/1 -> Add3/2
  Add3/1 -> [Te]
  [Te] -> Add4/1
  Constant1/1 -> Add4/2
  Add4/1 -> Gain4/1
  Gain3/1 -> Add4/3
  Constant3/1 -> Add5/2
  Add5/1 -> Gain3/1, [w]
  Constant6/1 -> Trigonometric Function3/1, Trigonometric Function2/1
  Trigonometric Function2/1 -> Gain5/1
  Trigonometric Function3/1 -> Gain6/1
  Gain5/1 -> Product2/1
  Gain6/1 -> Product3/2
  Gain8/1 -> [i_abc]
  Gain4/1 -> Integrator1/1, Discrete-Time Integrator1/1
  Voltage Measurement/1 -> Mux4/1
  Voltage Measurement1/1 -> Mux4/2
  Voltage Measurement2/1 -> Mux4/3
  Mux4/1 -> Gain11/1
  Gain11/1 -> [v_abc]
  Gain7/1 -> Demux/1
  Add/1 -> Math Function1/1
  Constant4/1 -> Math Function1/2
  Math Function1/1 -> [theta]
  [v_abc] -> abc->dq (Power-Invariant)1/1
  abc->dq (Power-Invariant)1/1 -> [v_dq]
  [w] -> Product3/1, Product2/2
  Constant5/1 -> Trigonometric Function/1, Trigonometric Function1/1
  Manual Switch1/1 -> Add5/1
  Constant10/1 -> Manual Switch1/1
  [theta] -> dq->abc (Power-Invariant)/2
  [theta] -> abc->dq (Power-Invariant)/2
  [theta] -> abc->dq (Power-Invariant)1/2
  [theta] -> Bus Creator/9  "theta"
  [e_dq] -> Bus Creator/4  "e_dq"
  [Te] -> Bus Creator/7  "Te"
  [i_abc] -> Bus Creator/3  "i_abc"
  [v_abc] -> Bus Creator/2  "v_abc"
  [v_dq] -> Bus Creator/5  "v_dq"
  [i_dq] -> Bus Creator/6  "i_dq"
  [e_abc] -> Bus Creator/1  "e_abc"
  [w] -> Bus Creator/8  "w"
  dq->abc (Power-Invariant)/1 -> [e_abc]
  Bus Creator/1 -> m/1
  Gain10/1 -> Discrete-Time Integrator/1, Integrator/1
  Integrator/1 -> Manual Switch2/2
  Manual Switch2/1 -> Add/1
  Discrete-Time Integrator/1 -> Manual Switch2/1
  Manual Switch3/1 -> Manual Switch1/2
  Integrator1/1 -> Manual Switch3/2
  Discrete-Time Integrator1/1 -> Manual Switch3/1
  connections:
  Current Measurement/RConn1 -- Winding A/RConn1
  Controlled Voltage Source/RConn1 -- Winding A/LConn1
  Current Measurement2/RConn1 -- Winding C/RConn1
  Current Measurement/LConn1 -- Voltage Measurement/LConn1 -- a/RConn1
  Current Measurement1/LConn1 -- Voltage Measurement1/LConn1 -- b/RConn1
  Current Measurement1/RConn1 -- Winding B/RConn1
  Winding B/LConn1 -- Controlled Voltage Source1/RConn1
  Controlled Voltage Source/LConn1 -- Voltage Measurement2/LConn2 -- Voltage Measurement1/LConn2 -- Voltage Measurement/LConn2 -- Controlled Voltage Source2/LConn1 -- n/RConn1 -- Controlled Voltage Source1/LConn1
  Winding C/LConn1 -- Controlled Voltage Source2/RConn1
  Current Measurement2/LConn1 -- Voltage Measurement2/LConn1 -- c/RConn1

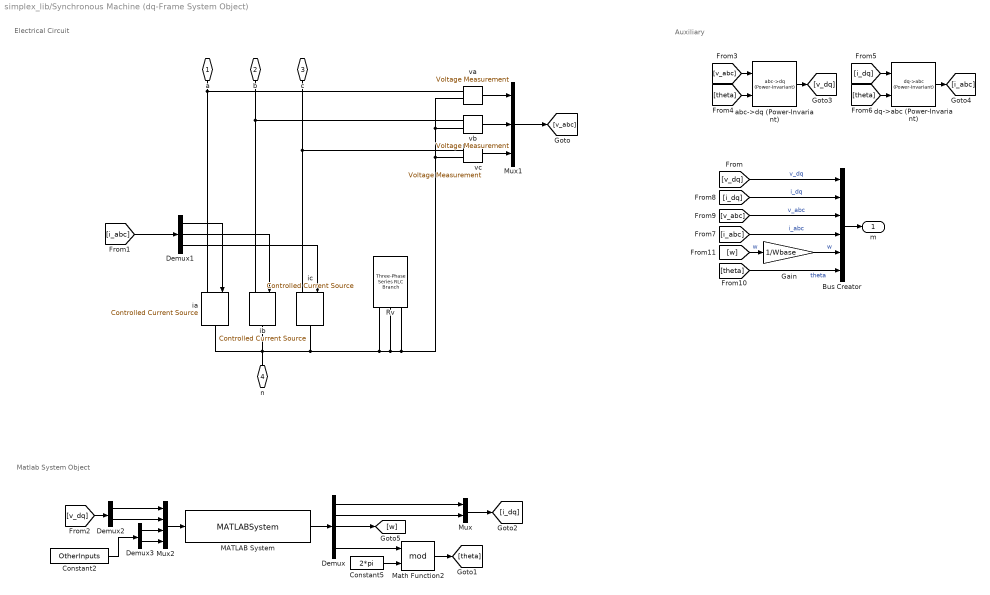
== system simplex_lib/Synchronous Machine (dq-Frame System Object) ==
  note: Matlab System Object
  note: Auxiliary
  note: Electrical Circuit
  Bus Creator : BusCreator  Inputs=6
  Constant2 : Constant  Value=OtherInputs
  Constant5 : Constant  Value=2*pi
  Demux : Demux  Outputs=5
  Demux1 : Demux  Outputs=3
  Demux2 : Demux  Outputs=2
  Demux3 : Demux  Outputs=2
  Gain : Gain  Gain=1/Wbase
  MATLAB System : MATLABSystem  System=Class_SynchronousMachine  DeviceType=DeviceType  Para=DevicePara  PowerFlow=PowerFlow  Ts=Ts  x0=x0  SimulateUsing=Code generation
      mask Type: Class_SynchronousMachine
      mask Display:
      | disp('Class_SynchronousMachine');
      | port_label('input',1,'u');
      | port_label('output',1,'y');
  Math Function2 : Math  Operator=mod  SignedPower=on  SaturateOnIntegerOverflow=on
  Mux : Mux  Inputs=2
  Mux1 : Mux  Inputs=3
  Mux2 : Mux
  Rv : powerlib/Elements/Three-Phase Series RLC Branch  LConnTagsString=A|B|C  RConnTagsString=A|B|C  BranchType=R  Resistance=2*DevicePara(3)/Ts  Inductance=1e-3  Capacitance=1e-6  Measurements=None
  abc->dq (Power-Invariant) : $bdroot/abc->dq (Power-Invariant)  SystemSampleTime=-1  VariantActivationTime=update diagram  Latency=0  AutoFrameSizeCalculation=off
  dq->abc (Power-Invariant) : $bdroot/dq->abc (Power-Invariant)  SystemSampleTime=-1  VariantActivationTime=update diagram  Latency=0  AutoFrameSizeCalculation=off
  ia : powerlib/Electrical Sources/Controlled Current Source  Initialize=on  Source_Type=AC  Amplitude=0  Phase=0  Frequency=0  Measurements=None
  ib : powerlib/Electrical Sources/Controlled Current Source  Initialize=on  Source_Type=AC  Amplitude=0  Phase=0  Frequency=0  Measurements=None
  ic : powerlib/Electrical Sources/Controlled Current Source  Initialize=on  Source_Type=AC  Amplitude=0  Phase=0  Frequency=0  Measurements=None
  va : powerlib/Measurements/Voltage Measurement  PhasorSimulation=off  OutputType=Complex  PSBequivalent=0
  vb : powerlib/Measurements/Voltage Measurement  PhasorSimulation=off  OutputType=Complex  PSBequivalent=0
  vc : powerlib/Measurements/Voltage Measurement  PhasorSimulation=off  OutputType=Complex  PSBequivalent=0
  a : PMIOPort  Side=Left
  b : PMIOPort  Port=2  Side=Left
  c : PMIOPort  Port=3  Side=Left
  n : PMIOPort  Port=4  Side=Left
  m : Outport
  wires:
  Demux/2 -> Mux/2
  Demux/1 -> Mux/1
  Mux/1 -> [i_dq]
  Demux/3 -> [w]
  Demux1/1 -> ia/1
  Demux1/2 -> ib/1
  va/1 -> Mux1/1
  vb/1 -> Mux1/2
  [v_dq] -> Demux2/1
  Demux2/1 -> Mux2/1
  Demux2/2 -> Mux2/2
  [v_abc] -> abc->dq (Power-Invariant)/1
  [theta] -> abc->dq (Power-Invariant)/2
  abc->dq (Power-Invariant)/1 -> [v_dq]
  [i_dq] -> dq->abc (Power-Invariant)/1
  [theta] -> dq->abc (Power-Invariant)/2
  dq->abc (Power-Invariant)/1 -> [i_abc]
  Mux2/1 -> MATLAB System/1
  MATLAB System/1 -> Demux/1
  vc/1 -> Mux1/3
  Demux1/3 -> ic/1
  Demux/5 -> Math Function2/1
  Constant5/1 -> Math Function2/2
  Math Function2/1 -> [theta]
  [v_dq] -> Bus Creator/1  "v_dq"
  [i_dq] -> Bus Creator/2  "i_dq"
  [v_abc] -> Bus Creator/3  "v_abc"
  [i_abc] -> Bus Creator/4  "i_abc"
  [w] -> Gain/1  "w"
  [theta] -> Bus Creator/6  "theta"
  Bus Creator/1 -> m/1
  Gain/1 -> Bus Creator/5  "w"
  Mux1/1 -> [v_abc]
  Constant2/1 -> Demux3/1
  Demux3/1 -> Mux2/3
  Demux3/2 -> Mux2/4
  [i_abc] -> Demux1/1
  connections:
  vb/LConn2 -- va/LConn2 -- vc/LConn2 -- Rv/RConn3 -- Rv/RConn2 -- Rv/RConn1 -- ia/RConn1 -- ib/RConn1 -- n/RConn1 -- ic/RConn1
  a/RConn1 -- ia/LConn1 -- va/LConn1
  b/RConn1 -- ib/LConn1 -- vb/LConn1
  vc/LConn1 -- ic/LConn1 -- c/RConn1

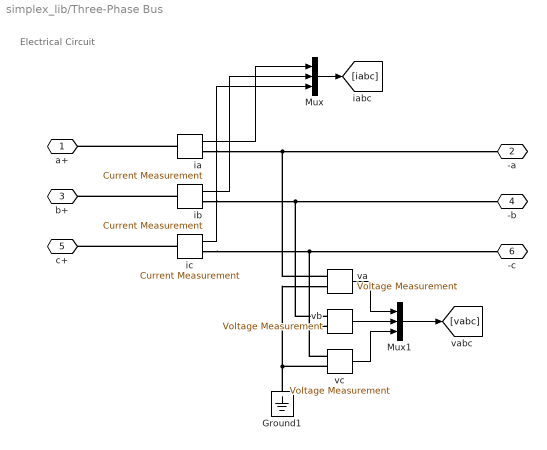
== system simplex_lib/Three-Phase Bus ==
  note: Electrical Circuit
  Ground1 : powerlib/Elements/Ground  LConnTagsString=a
  Mux : Mux  Inputs=3
  Mux1 : Mux  Inputs=3
  ia : powerlib/Measurements/Current Measurement  PhasorSimulation=off  OutputType=Complex  PSBequivalent=0
  ib : powerlib/Measurements/Current Measurement  PhasorSimulation=off  OutputType=Complex  PSBequivalent=0
  ic : powerlib/Measurements/Current Measurement  PhasorSimulation=off  OutputType=Complex  PSBequivalent=0
  va : powerlib/Measurements/Voltage Measurement  PhasorSimulation=off  OutputType=Complex  PSBequivalent=0
  vb : powerlib/Measurements/Voltage Measurement  PhasorSimulation=off  OutputType=Complex  PSBequivalent=0
  vc : powerlib/Measurements/Voltage Measurement  PhasorSimulation=off  OutputType=Complex  PSBequivalent=0
  a+ : PMIOPort  Side=Left
  -a : PMIOPort  Port=2  Side=Right
  b+ : PMIOPort  Port=3  Side=Left
  -b : PMIOPort  Port=4  Side=Right
  c+ : PMIOPort  Port=5  Side=Left
  -c : PMIOPort  Port=6  Side=Right
  wires:
  Mux/1 -> [iabc]
  ia/1 -> Mux/1
  ib/1 -> Mux/2
  ic/1 -> Mux/3
  vb/1 -> Mux1/2
  va/1 -> Mux1/1
  vc/1 -> Mux1/3
  Mux1/1 -> [vabc]
  connections:
  ic/RConn1 -- vc/LConn1 -- -c/RConn1
  ib/LConn1 -- b+/RConn1
  ib/RConn1 -- vb/LConn1 -- -b/RConn1
  ic/LConn1 -- c+/RConn1
  ia/LConn1 -- a+/RConn1
  ia/RConn1 -- va/LConn1 -- -a/RConn1
  Ground1/LConn1 -- vc/LConn2 -- vb/LConn2 -- va/LConn2

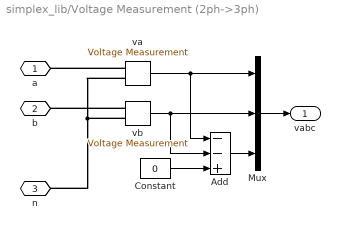
== system simplex_lib/Voltage Measurement (2ph->3ph) ==
  Add : Sum  Inputs=--+
  Constant : Constant  Value=0
  Mux : Mux  Inputs=3
  va : powerlib/Measurements/Voltage Measurement  PhasorSimulation=off  OutputType=Complex  PSBequivalent=0
  vb : powerlib/Measurements/Voltage Measurement  PhasorSimulation=off  OutputType=Complex  PSBequivalent=0
  a : PMIOPort  Side=Left
  b : PMIOPort  Port=2  Side=Left
  n : PMIOPort  Port=3  Side=Left
  vabc : Outport
  wires:
  Mux/1 -> vabc/1
  va/1 -> Mux/1, Add/1
  vb/1 -> Mux/2, Add/2
  Constant/1 -> Add/3
  Add/1 -> Mux/3
  connections:
  vb/LConn2 -- va/LConn2 -- n/RConn1
  vb/LConn1 -- b/RConn1
  va/LConn1 -- a/RConn1

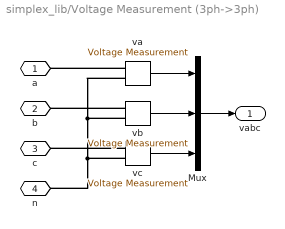
== system simplex_lib/Voltage Measurement (3ph->3ph) ==
  Mux : Mux  Inputs=3
  va : powerlib/Measurements/Voltage Measurement  PhasorSimulation=off  OutputType=Complex  PSBequivalent=0
  vb : powerlib/Measurements/Voltage Measurement  PhasorSimulation=off  OutputType=Complex  PSBequivalent=0
  vc : powerlib/Measurements/Voltage Measurement  PhasorSimulation=off  OutputType=Complex  PSBequivalent=0
  a : PMIOPort  Side=Left
  b : PMIOPort  Port=2  Side=Left
  c : PMIOPort  Port=3  Side=Left
  n : PMIOPort  Port=4  Side=Left
  vabc : Outport
  wires:
  vc/1 -> Mux/3
  Mux/1 -> vabc/1
  va/1 -> Mux/1
  vb/1 -> Mux/2
  connections:
  vb/LConn2 -- va/LConn2 -- vc/LConn2 -- n/RConn1
  vc/LConn1 -- c/RConn1
  vb/LConn1 -- b/RConn1
  va/LConn1 -- a/RConn1

== system simplex_lib/abc->alpha//beta (Power-Invariant) ==
  abc : Inport
  ->alpha : Fcn  Expr=u(1) - 1/2*u(2) - 1/2*u(3)
  ->beta : Fcn  Expr=0 + sqrt(3)/2*u(2) - sqrt(3)/2*u(3)
  Gain : Gain  Gain=sqrt(2/3)
  Mux2 : Mux  Inputs=2
  albe : Outport  VectorParamsAs1DForOutWhenUnconnected=off
  wires:
  abc/1 -> Gain/1
  Mux2/1 -> albe/1
  Gain/1 -> ->alpha/1, ->beta/1
  ->alpha/1 -> Mux2/1
  ->beta/1 -> Mux2/2

== system simplex_lib/abc->alpha//beta//0 (Power-Invariant) ==
  abc : Inport
  ->0 : Fcn  Expr=1/sqrt(2)*u(1) + 1/sqrt(2)*u(2) + 1/sqrt(2)*u(3)
  ->alpha : Fcn  Expr=u(1) - 1/2*u(2) - 1/2*u(3)
  ->beta : Fcn  Expr=0 + sqrt(3)/2*u(2) - sqrt(3)/2*u(3)
  Gain : Gain  Gain=sqrt(2/3)
  Mux2 : Mux  Inputs=3
  albe0 : Outport
  wires:
  ->beta/1 -> Mux2/2
  ->alpha/1 -> Mux2/1
  Gain/1 -> ->alpha/1, ->0/1, ->beta/1
  Mux2/1 -> albe0/1
  abc/1 -> Gain/1
  ->0/1 -> Mux2/3

== system simplex_lib/abc->dq (Power-Invariant) ==
  abc : Inport
  theta : Inport  Port=2
  ->d : Fcn  Expr=cos(u(4))*u(1) + cos(u(4)-2/3*pi)*u(2) + cos(u(4)-4/3*pi)*u(3)
  ->q : Fcn  Expr=-sin(u(4))*u(1) - sin(u(4)-2/3*pi)*u(2) - sin(u(4)-4/3*pi)*u(3)
  Gain : Gain  Gain=sqrt(2/3)
  Mux5 : Mux  Inputs=2
  Mux6 : Mux  Inputs=2
  dq : Outport
  wires:
  Mux5/1 -> ->q/1, ->d/1
  Mux6/1 -> dq/1
  ->q/1 -> Mux6/2
  theta/1 -> Mux5/2
  Gain/1 -> Mux5/1
  ->d/1 -> Mux6/1
  abc/1 -> Gain/1

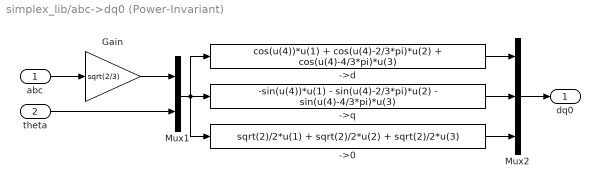
== system simplex_lib/abc->dq0 (Power-Invariant) ==
  abc : Inport
  theta : Inport  Port=2
  ->0 : Fcn  Expr=sqrt(2)/2*u(1) + sqrt(2)/2*u(2) + sqrt(2)/2*u(3)
  ->d : Fcn  Expr=cos(u(4))*u(1) + cos(u(4)-2/3*pi)*u(2) + cos(u(4)-4/3*pi)*u(3)
  ->q : Fcn  Expr=-sin(u(4))*u(1) - sin(u(4)-2/3*pi)*u(2) - sin(u(4)-4/3*pi)*u(3)
  Gain : Gain  Gain=sqrt(2/3)
  Mux1 : Mux  Inputs=2
  Mux2 : Mux  Inputs=3
  dq0 : Outport
  wires:
  ->d/1 -> Mux2/1
  ->q/1 -> Mux2/2
  Gain/1 -> Mux1/1
  abc/1 -> Gain/1
  theta/1 -> Mux1/2
  Mux1/1 -> ->0/1, ->d/1, ->q/1
  Mux2/1 -> dq0/1
  ->0/1 -> Mux2/3

== system simplex_lib/alpha//beta->abc (Power-Invariant) ==
  albe : Inport
  ->a : Fcn  Expr=u(1) + 0
  ->b : Fcn  Expr=-1/2*u(1) + sqrt(3)/2*u(2)
  ->c : Fcn  Expr=-1/2*u(1) - sqrt(3)/2*u(2)
  Gain : Gain  Gain=sqrt(2/3)
  Mux2 : Mux  Inputs=3
  abc : Outport
  wires:
  Gain/1 -> ->a/1, ->c/1, ->b/1
  Mux2/1 -> abc/1
  ->c/1 -> Mux2/3
  ->b/1 -> Mux2/2
  ->a/1 -> Mux2/1
  albe/1 -> Gain/1

== system simplex_lib/alpha//beta//0->abc (Power-Invariant) ==
  albe0 : Inport
  ->a : Fcn  Expr=u(1) + 0 + 1/sqrt(2)*u(3)
  ->b : Fcn  Expr=-1/2*u(1) + sqrt(3)/2*u(2) + 1/sqrt(2)*u(3)
  ->c : Fcn  Expr=-1/2*u(1) - sqrt(3)/2*u(2) + 1/sqrt(2)*u(3)
  Gain : Gain  Gain=sqrt(2/3)
  Mux2 : Mux  Inputs=3
  abc : Outport
  wires:
  Gain/1 -> ->a/1, ->c/1, ->b/1
  ->c/1 -> Mux2/3
  albe0/1 -> Gain/1
  ->a/1 -> Mux2/1
  ->b/1 -> Mux2/2
  Mux2/1 -> abc/1

== system simplex_lib/dq->abc (Power-Invariant) ==
  dq : Inport
  theta : Inport  Port=2
  ->a : Fcn  Expr=cos(u(3))*u(1) - sin(u(3))*u(2)
  ->b : Fcn  Expr=cos(u(3)-2/3*pi)*u(1) - sin(u(3)-2/3*pi)*u(2)
  ->c : Fcn  Expr=cos(u(3)-4/3*pi)*u(1) - sin(u(3)-4/3*pi)*u(2)
  Gain : Gain  Gain=sqrt(2/3)
  Mux5 : Mux  Inputs=2
  Mux6 : Mux  Inputs=3
  abc : Outport
  wires:
  theta/1 -> Mux5/2
  Mux5/1 -> ->c/1, ->a/1, ->b/1
  Mux6/1 -> abc/1
  ->c/1 -> Mux6/3
  dq/1 -> Gain/1
  Gain/1 -> Mux5/1
  ->a/1 -> Mux6/1
  ->b/1 -> Mux6/2

== system simplex_lib/dq0->abc (Power-Invariant) ==
  dq0 : Inport
  theta : Inport  Port=2
  ->a : Fcn  Expr=cos(u(4))*u(1) - sin(u(4))*u(2) + sqrt(2)/2*u(3)
  ->b : Fcn  Expr=cos(u(4)-2/3*pi)*u(1) - sin(u(4)-2/3*pi)*u(2) + sqrt(2)/2*u(3)
  ->c : Fcn  Expr=cos(u(4)-4/3*pi)*u(1) - sin(u(4)-4/3*pi)*u(2) + sqrt(2)/2*u(3)
  Gain : Gain  Gain=sqrt(2/3)
  Mux1 : Mux  Inputs=2
  Mux2 : Mux  Inputs=3
  abc : Outport
  wires:
  ->a/1 -> Mux2/1
  ->b/1 -> Mux2/2
  Gain/1 -> Mux1/1
  dq0/1 -> Gain/1
  theta/1 -> Mux1/2
  Mux1/1 -> ->c/1, ->a/1, ->b/1
  Mux2/1 -> abc/1
  ->c/1 -> Mux2/3
